simulink model "controller_simulator"  (R2025b)
settings: Solver=VariableStepAuto  StartTime=0.0  StopTime=1000  RelTol=1e-3
values from neighbouring files (symbols this model uses):
  FO_PI = minreal(kp_FO + kp_FO*ki_FO*tf(1,[1 0])*s_alfa1, 0.1)    [controller_design.m]
  Hc_GT = minreal((1/H_p) * (Ho_GT / (1-Ho_GT)))    [controller_design.m]
  Hc_PI = minreal(ki_PI * (1 + tf(1, [Ti_PI 0])))    [controller_design.m]
  Rc_IMC = minreal(Hc_IMC / minreal(1 - Hc_IMC * H_p))    [controller_design.m]
undefined symbols (not defined in the file or in its folder): MAP_model, paramGrecoMAP
libraries: slpidlib x1
settings Model: Creator=ciuba  LastModifiedBy=ciuba

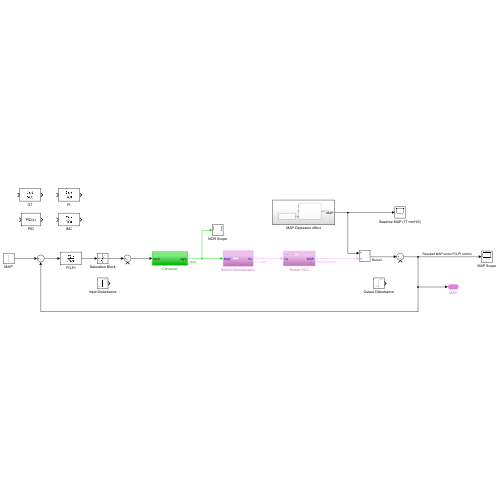
[thumbnail: Simulink's stored preview of the top-level diagram]
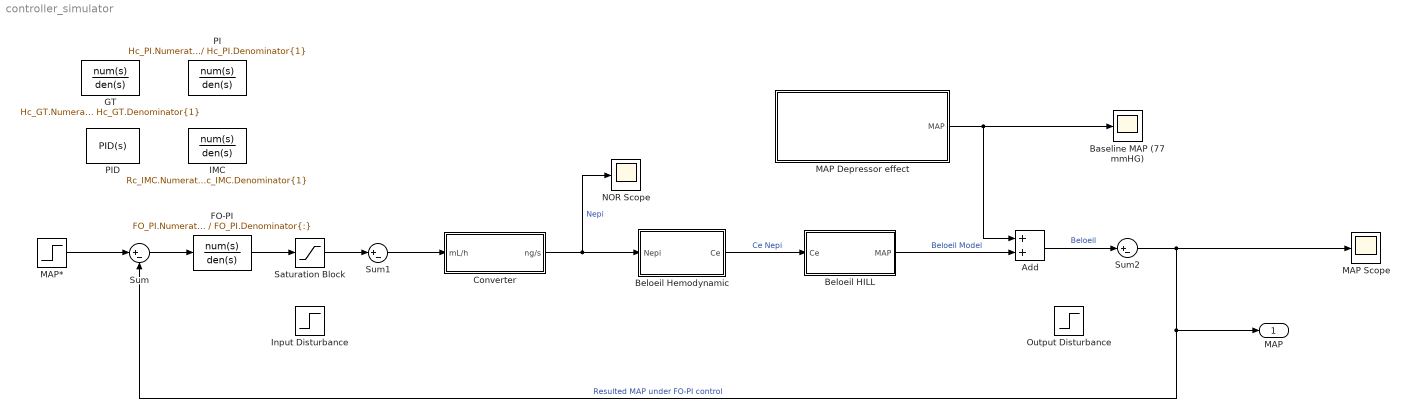
== system controller_simulator ==
  Add : Sum
  Baseline MAP (77 mmHG) : Scope
      settings: ActiveDisplayYMinimum=-1  ActiveDisplayYMaximum=1  DataLoggingVariableName=ScopeData6
  Beloeil HILL : Subsystem
  Beloeil Hemodynamic : Subsystem
  Converter : Subsystem
  FO-PI : TransferFcn  Numerator=FO_PI.Numerator{:}  Denominator=FO_PI.Denominator{:}
  GT : TransferFcn  Numerator=Hc_GT.Numerator{1}  Denominator=Hc_GT.Denominator{1}
  IMC : TransferFcn  Numerator=Rc_IMC.Numerator{1}  Denominator=Rc_IMC.Denominator{1}
  Input Disturbance : Step  Time=500  After=50  SampleTime=0
  MAP Depressor effect : Subsystem
  MAP Scope : Scope
      settings: ActiveDisplayYMinimum=75.219588427113237  ActiveDisplayYMaximum=93.023704155980838  DataLoggingVariableName=ScopeData4
  MAP* : Step  After=90  SampleTime=0
  NOR Scope : Scope
      settings: ActiveDisplayYMinimum=-446.02327911069489  ActiveDisplayYMaximum=4014.2095119962551  DataLoggingVariableName=ScopeData10  DataLoggingSaveFormat=Array
  Output Disturbance : Step  Time=500  After=5  SampleTime=0
  PI : TransferFcn  Numerator=Hc_PI.Numerator{1}  Denominator=Hc_PI.Denominator{1}
  PID : slpidlib/PID Controller  Controller=PID  Form=Parallel  TimeDomain=Continuous-time  UseExternalTs=off  SampleTime=-1  IntegratorMethod=Forward Euler  FilterMethod=Forward Euler  ControllerParametersSource=internal  P=35.6  I=4.93  UseKiTs=off  D=64.4  UseExternalDerivativeSource=off  N=100  UseFilter=on  TunerSelectOption=Transfer Function Based (PID Tuner App)  InitialConditionSource=internal  InitialConditionForIntegrator=0  InitialConditionForFilter=0  DifferentiatorICPrevScaledInput=0  ExternalReset=none  TrackingMode=off  Kt=1  LimitOutput=off  SatLimitsSource=internal  UpperSaturationLimit=inf  LowerSaturationLimit=-inf  LinearizeAsGain=on  AntiWindupMode=none  Kb=1  LimitIntegrator=off  UpperIntegratorSaturationLimit=inf  LowerIntegratorSaturationLimit=-inf  POutMin=[]  POutMax=[]  IOutMin=[]  IOutMax=[]  DOutMin=[]  DOutMax=[]  NOutMin=[]  NOutMax=[]  SumOutMin=[]  SumOutMax=[]  SaturationOutMin=[]  SaturationOutMax=[]  PParamMin=[]  PParamMax=[]  IParamMin=[]  IParamMax=[]  DParamMin=[]  DParamMax=[]  NParamMin=[]  NParamMax=[]  KbParamMin=[]  KbParamMax=[]  KtParamMin=[]  KtParamMax=[]  KbOutMin=[]  KbOutMax=[]  KtOutMin=[]  KtOutMax=[]  IntegratorOutMin=[]  IntegratorOutMax=[]  FilterOutMin=[]  FilterOutMax=[]  SumI1OutMin=[]  SumI1OutMax=[]  SumI2OutMin=[]  SumI2OutMax=[]  SumI3OutMin=[]  SumI3OutMax=[]  SumI4OutMin=[]  SumI4OutMax=[]  SumDOutMin=[]  SumDOutMax=[]  DifferentiatorOutMin=[]  DifferentiatorOutMax=[]  FilterDiffOutCoefMin=[]  FilterDiffOutCoefMax=[]  ReciprocalOutMin=[]  ReciprocalOutMax=[]  SumDenOutMin=[]  SumDenOutMax=[]  SumNumOutMin=[]  SumNumOutMax=[]  DivideOutMin=[]  DivideOutMax=[]  UdiffTsProdOutMin=[]  UdiffTsProdOutMax=[]  NTsProdOutMin=[]  NTsProdOutMax=[]  UintegralTsProdOutMin=[]  UintegralTsProdOutMax=[]  UngainTsProdOutMin=[]  UngainTsProdOutMax=[]  ClampingZeroOutDataTypeStr=Inherit: Inherit via back propagation  ClampingZeroOutMin=[]  ClampingZeroOutMax=[]  FilterDenConstantOutDataTypeStr=Inherit: Inherit via back propagation  FilterDenConstantOutMin=[]  FilterDenConstantOutMax=[]  PCopyOutDataTypeStr=Inherit: Inherit via back propagation  PCopyOutMin=[]  PCopyOutMax=[]  NCopyOutDataTypeStr=Inherit: Inherit via back propagation  NCopyOutMin=[]  NCopyOutMax=[]  IntegratorContinuousStateAttributes=''  IntegratorStateMustResolveToSignalObject=off  IntegratorRTWStateStorageClass=Auto  FilterContinuousStateAttributes=''  FilterStateMustResolveToSignalObject=off  FilterRTWStateStorageClass=Auto  ParallelPVariant=InternalParameters  IdealPVariant=Disabled  IVariant=InternalParameters  DVariant=InternalParameters  IntegratorVariant=Continuous  SatVariant=Disabled  AWVariant=Passthrough  PCopyVariant=Disabled  TRVariant=Disabled  FdbkBlocksVariant=Forward  IdealPFdbkVariant=Disabled  SatFdbkVariant=Disabled  DerivativeFilterVariant=ContFilter  NVariant=InternalParameters  NCopyVariant=Disabled  FilterICVariant=InternalICsFilter  IntegratorICVariant=InternalICs  ExternalResetVariant=Disabled  TRSumVariant=Passthrough  SumFdbkVariant=Disabled  SumVariant=Sum_PID  TsampFilterVariant=InternalTs  TsampNgainVariant=Passthrough  TsampIntegralVariant=Disabled_SignalSpec  ExternalSaturationOutDataTypeStr=Inherit: Same as second input  DerivativeSourceVariant=ErrorSignal  PreIntVariant=InternalPreInt
  Saturation Block : Saturate  UpperLimit=5000  LowerLimit=0
  Sum : Sum  Inputs=|+-
  Sum1 : Sum  Inputs=|+-
  Sum2 : Sum  Inputs=|+-
  MAP : Outport
  wires:
  Sum/1 -> FO-PI/1
  MAP*/1 -> Sum/1
  Beloeil HILL/1(MAP) -> Add/2  "Beloeil Model"
  Sum1/1 -> Converter/1(mL/h)
  MAP Depressor effect/1(MAP) -> Add/1, Baseline MAP (77 mmHG)/1
  FO-PI/1 -> Saturation Block/1
  Saturation Block/1 -> Sum1/1
  Converter/1(ng/s) -> NOR Scope/1, Beloeil Hemodynamic/1(Nepi)  "Nepi"
  Beloeil Hemodynamic/1(Ce) -> Beloeil HILL/1(Ce)  "Ce Nepi"
  Add/1 -> Sum2/1  "Beloeil"
  Sum2/1 -> Sum/2, MAP/1, MAP Scope/1  "Resulted MAP under FO-PI control"

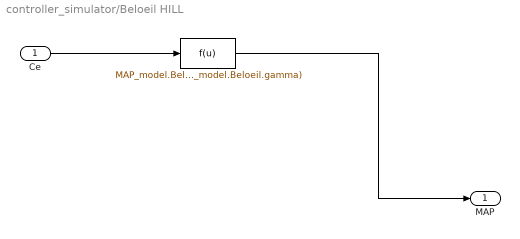
== system controller_simulator/Beloeil HILL ==
  Ce : Inport
  " " : Fcn  Expr=MAP_model.Beloeil.Emax * (u^MAP_model.Beloeil.gamma) / (MAP_model.Beloeil.EC50^MAP_model.Beloeil.gamma+u^MAP_model.Beloeil.gamma)
  MAP : Outport
  wires:
  " "/1 -> MAP/1
  Ce/1 -> " "/1

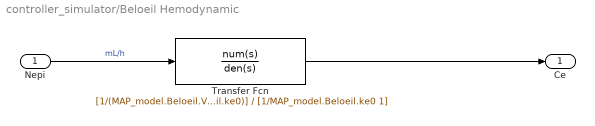
== system controller_simulator/Beloeil Hemodynamic ==
  Nepi : Inport
  Transfer Fcn : TransferFcn  Numerator=[1/(MAP_model.Beloeil.Vd*MAP_model.Beloeil.ke0)]  Denominator=[1/MAP_model.Beloeil.ke0 1]
  Ce : Outport
  wires:
  Nepi/1 -> Transfer Fcn/1  "mL/h"
  Transfer Fcn/1 -> Ce/1

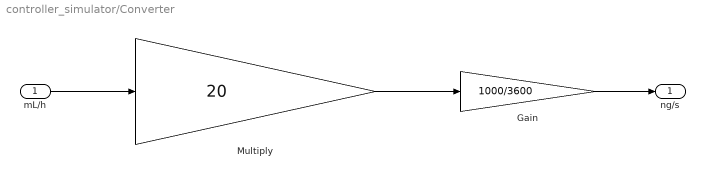
== system controller_simulator/Converter ==
  mL/h : Inport
  Gain : Gain  Gain=1000/3600
  Multiply : Gain  Gain=20
  ng/s : Outport
  wires:
  Gain/1 -> ng/s/1
  Multiply/1 -> Gain/1
  mL/h/1 -> Multiply/1

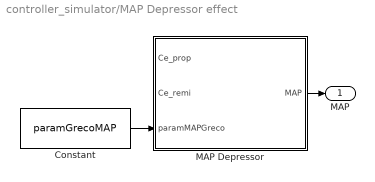
== system controller_simulator/MAP Depressor effect ==
  Constant : Constant  Value=paramGrecoMAP  OutDataTypeStr=Bus: GrecoMAPBus
  MAP Depressor : MATLAB Function  TreatAsAtomicUnit=on
  MAP : Outport
  wires:
  MAP Depressor/1(MAP) -> MAP/1
  Constant/1 -> MAP Depressor/3(paramMAPGreco)

== matlab function controller_simulator/MAP Depressor effect/MAP Depressor ==
  data: Ce_prop input; MAP output; Ce_remi input; paramMAPGreco input
function MAP = MAP_Greco(Ce_prop, Ce_remi, paramMAPGreco)    
    % Extract parameters from bus
    C50P   = paramMAPGreco.Prop.C50;    % Propofol EC50 (μg/mL)
    gammaP = paramMAPGreco.Prop.gamma;  % Propofol Hill
    C50R   = paramMAPGreco.Remi.C50;    % Remifentanil EC50 (ng/mL)
    gammaR = paramMAPGreco.Remi.gamma;  % Remifentanil Hill
    alpha  = paramMAPGreco.Interaction.alpha;  % Synergy parameter
    Emax   = paramMAPGreco.Interaction.Emax;   % Max MAP depression (mmHg)
    MAP0   = paramMAPGreco.Interaction.MAP0;   % Baseline MAP (mmHg)
    
    % Compute normalized concentrations
    X = (Ce_prop / C50P)^gammaP;
    Y = (Ce_remi / C50R)^gammaR;
    
    % Numerator/denominator as per Greco response surface
    numerator   = X + Y + alpha * X * Y;
    denominator = 1 + X + Y + alpha * X * Y;
    MAP_depr    = Emax * numerator / denominator;
    
    % Net MAP (subtract depressant effect from baseline)
    MAP = MAP0 - MAP_depr;
end
